simulink model "CraneController"  (R2020b)
settings: Solver=ode45  StartTime=0.0  StopTime=10  MaxStep=1e-5  RelTol=1e-4
values from neighbouring files (symbols this model uses):
  c1 = -3    [ThongSo.m]    (also in ThongSo_Change.m)
  c2 = -3    [ThongSo.m]    (also in ThongSo_Change.m)
  c3 = 10.3    [ThongSo.m]    (also in ThongSo_Change.m)
  c4 = 1    [ThongSo.m]    (also in ThongSo_Change.m)
  eta = 0.05    [ThongSo.m]    (also in ThongSo_Change.m)
  g = 9.81    [ThongSo.m]    (also in ThongSo_Change.m)
  L = 0.305    [ThongSo.m]    (also in ThongSo_Change.m = 0.8)
  M = 1    [ThongSo.m]    (also in ThongSo_Change.m = 5)
  m = 0.8    [ThongSo.m]    (also in ThongSo_Change.m = 1.5)
  tau = 4    [ThongSo.m]    (also in ThongSo_Change.m)
  theta0 = 0    [ThongSo.m]    (also in ThongSo_Change.m)
  theta0_dot = 0    [ThongSo.m]    (also in ThongSo_Change.m)
  theta0_dotdot = 0    [ThongSo.m]    (also in ThongSo_Change.m)
  thetad = 0    [ThongSo.m]    (also in ThongSo_Change.m)
  thetad_dot = 0    [ThongSo.m]    (also in ThongSo_Change.m)
  x0 = 0    [ThongSo.m]    (also in ThongSo_Change.m)
  x0_dot = 0    [ThongSo.m]    (also in ThongSo_Change.m)
  x0_dotdot = 0    [ThongSo.m]    (also in ThongSo_Change.m)
  xd = 1    [ThongSo.m]    (also in ThongSo_Change.m = 2)
  xd_dot = 0    [ThongSo.m]    (also in ThongSo_Change.m)
libraries: powerlib x1
settings Model: Creator=chemi  LastModifiedBy=chemi
settings SolverCC: ZeroCrossAlgorithm=Adaptive
settings DebuggingCC: IgnoredZcDiagnostic=none

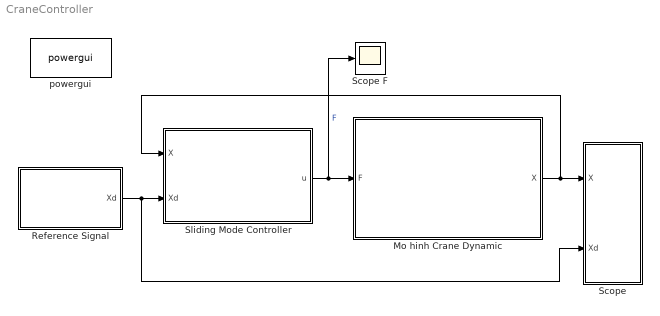
== system CraneController ==
  Mo hinh Crane Dynamic : Subsystem
  Reference Signal : Subsystem
  Scope : Subsystem
  Scope F : Scope
  Sliding Mode Controller : Subsystem
  powergui : powerlib/powergui  Priority=1  SimulationMode=Continuous  SampleTime=50e-6  frequency=60  Iterations=50  frequencyindice=60  Pbase=100e6  ErrMax=1e-4  UnitsV=kV  UnitsW=MW  buscounter=0  FunctionMessages=off  echomessages=off  EnableUseOfTLC=off  CurrentSourceSwitches=off  DisableSnubberDevices=off  DisableRonSwitches=off  DisableVfSwitches=off  DisplayEquations=off  AutomaticDiscreteSolvers=off  SolverType=Tustin/Backward Euler (TBE)  Interpol=off  ExternalGateDelay=off  methode=off  Ts=100  x0status=blocks  SPID=on  SwTol=0  HookPort=off  NonlinearTolerance=1e-4  nMaxIteration=100  ContinueOnMaxIteration=off  RestoreLinks=warning  ResistiveCurrentMeasurement=off  Frange=[0:2:500]  Ylog=off  Xlog=on  ShowGrid=off  save=off  variable=ZData  structure=0  ZoomFFT=off  StartTime=0.0  cycles=1  DisplayStyle=1  fundamental=60  FreqAxis=off  MaxFrequency=1000  frequencyindicesteady=1  RmsSteady=1  display=off
  wires:
  Reference Signal/1(Xd) -> Scope/2(Xd), Sliding Mode Controller/2(Xd)
  Sliding Mode Controller/1(u) -> Scope F/1, Mo hinh Crane Dynamic/1(F)  "F"
  Mo hinh Crane Dynamic/1(X) -> Sliding Mode Controller/1(X), Scope/1(X)

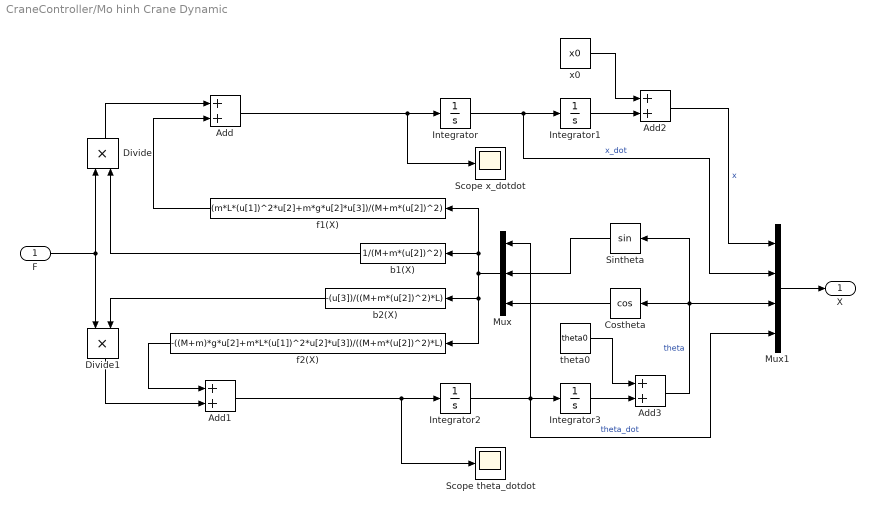
== system CraneController/Mo hinh Crane Dynamic ==
  F : Inport
  Add{,1..3} (4 alike) : Sum
  Costheta : Trigonometry  Operator=cos
  Divide : Product  Inputs=**
  Divide1 : Product  Inputs=**
  Integrator : Integrator  InitialCondition=x0_dotdot
  Integrator1 : Integrator  InitialCondition=x0_dot
  Integrator2 : Integrator  InitialCondition=theta0_dotdot
  Integrator3 : Integrator  InitialCondition=theta0_dot
  Mux : Mux  Inputs=3
  Mux1 : Mux
  Scope theta_dotdot : Scope
  Scope x_dotdot : Scope
  Sintheta : Trigonometry
  b1(X) : Fcn  Expr=1/(M+m*(u[2])^2)
  b2(X) : Fcn  Expr=-(u[3])/((M+m*(u[2])^2)*L)
  f1(X) : Fcn  Expr=(m*L*(u[1])^2*u[2]+m*g*u[2]*u[3])/(M+m*(u[2])^2)
  f2(X) : Fcn  Expr=-((M+m)*g*u[2]+m*L*(u[1])^2*u[2]*u[3])/((M+m*(u[2])^2)*L)
  theta0 : Constant  Value=theta0
  x0 : Constant  Value=x0
  X : Outport
  wires:
  Integrator1/1 -> Add2/2
  Integrator/1 -> Mux1/2, Integrator1/1  "x_dot"
  Integrator2/1 -> Mux1/4, Mux/1, Integrator3/1  "theta_dot"
  F/1 -> Divide/1, Divide1/1
  Mux/1 -> f1(X)/1, b1(X)/1, b2(X)/1, f2(X)/1
  Add/1 -> Scope x_dotdot/1, Integrator/1
  b1(X)/1 -> Divide/2
  Add1/1 -> Scope theta_dotdot/1, Integrator2/1
  f2(X)/1 -> Add1/1
  Divide1/1 -> Add1/2
  b2(X)/1 -> Divide1/2
  Divide/1 -> Add/1
  f1(X)/1 -> Add/2
  x0/1 -> Add2/1
  Integrator3/1 -> Add3/2
  theta0/1 -> Add3/1
  Add3/1 -> Mux1/3, Sintheta/1, Costheta/1  "theta"
  Sintheta/1 -> Mux/2
  Costheta/1 -> Mux/3
  Add2/1 -> Mux1/1  "x"
  Mux1/1 -> X/1

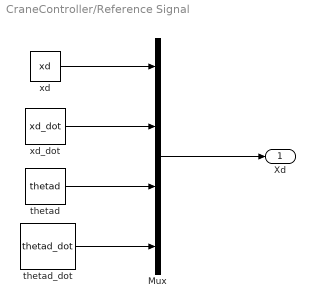
== system CraneController/Reference Signal ==
  Mux : Mux
  thetad : Constant  Value=thetad
  thetad_dot : Constant  Value=thetad_dot
  xd : Constant  Value=xd
  xd_dot : Constant  Value=xd_dot
  Xd : Outport
  wires:
  Mux/1 -> Xd/1
  thetad_dot/1 -> Mux/4
  xd/1 -> Mux/1
  xd_dot/1 -> Mux/2
  thetad/1 -> Mux/3

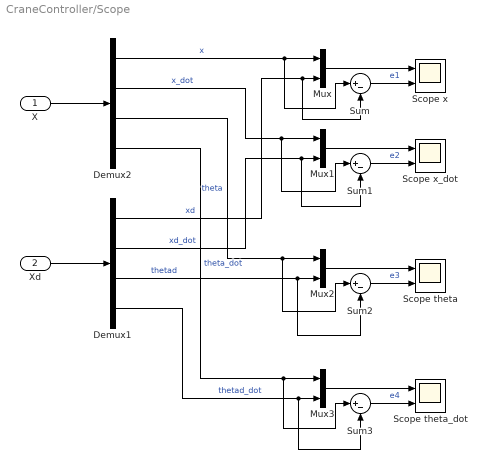
== system CraneController/Scope ==
  X : Inport
  Xd : Inport  Port=2
  Demux1 : Demux
  Demux2 : Demux
  Mux{,1..3} (4 alike) : Mux  Inputs=2
  Scope theta : Scope  NumInputPorts=2
  Scope theta_dot : Scope  NumInputPorts=2
  Scope x : Scope  NumInputPorts=2
  Scope x_dot : Scope  NumInputPorts=2
  Sum{,1..3} (4 alike) : Sum  Inputs=|+-
  wires:
  Mux/1 -> Scope x/1
  X/1 -> Demux2/1
  Xd/1 -> Demux1/1
  Demux2/1 -> Sum/1, Mux/1  "x"
  Demux1/1 -> Sum/2, Mux/2  "xd"
  Sum/1 -> Scope x/2  "e1"
  Demux2/2 -> Mux1/1, Sum1/1  "x_dot"
  Demux1/2 -> Mux1/2, Sum1/2  "xd_dot"
  Mux1/1 -> Scope x_dot/1
  Sum1/1 -> Scope x_dot/2  "e2"
  Demux2/3 -> Sum2/1, Mux2/1  "theta"
  Demux1/3 -> Sum2/2, Mux2/2  "thetad"
  Mux2/1 -> Scope theta/1
  Sum2/1 -> Scope theta/2  "e3"
  Demux2/4 -> Sum3/1, Mux3/1  "theta_dot"
  Demux1/4 -> Sum3/2, Mux3/2  "thetad_dot"
  Mux3/1 -> Scope theta_dot/1
  Sum3/1 -> Scope theta_dot/2  "e4"

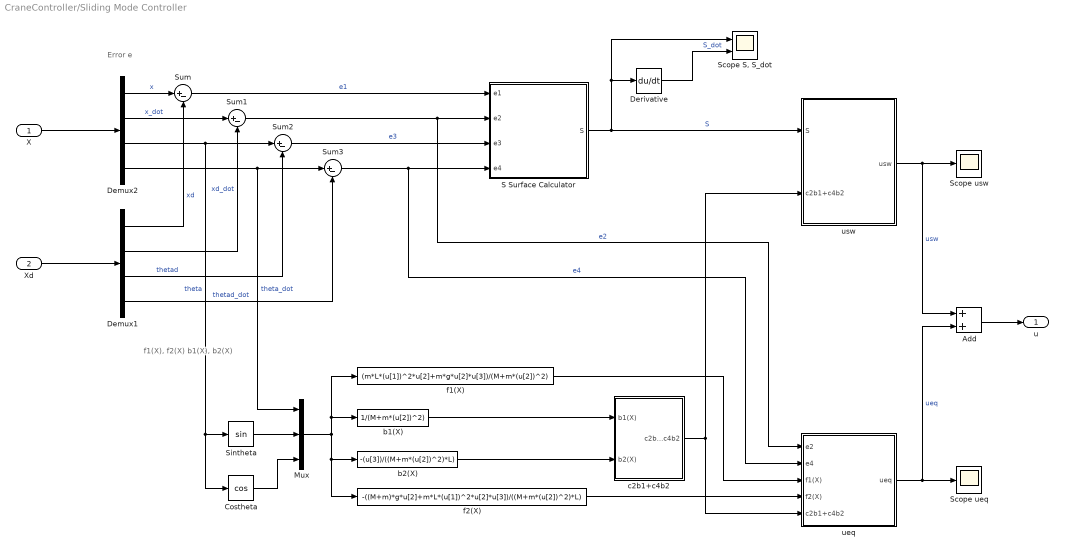
== system CraneController/Sliding Mode Controller ==
  note: Error e
  note: f1(X), f2(X)
      | b1(X), b2(X)
  X : Inport
  Xd : Inport  Port=2
  Add : Sum
  Costheta : Trigonometry  Operator=cos
  Demux1 : Demux
  Demux2 : Demux
  Derivative : Derivative
  Mux : Mux  Inputs=3
  S Surface Calculator : Subsystem
  "Scope S, S_dot" : Scope  NumInputPorts=2
  Scope ueq : Scope
  Scope usw : Scope
  Sintheta : Trigonometry
  Sum{,1..3} (4 alike) : Sum  Inputs=|+-
  b1(X) : Fcn  Expr=1/(M+m*(u[2])^2)
  b2(X) : Fcn  Expr=-(u[3])/((M+m*(u[2])^2)*L)
  c2b1+c4b2 : Subsystem
  f1(X) : Fcn  Expr=(m*L*(u[1])^2*u[2]+m*g*u[2]*u[3])/(M+m*(u[2])^2)
  f2(X) : Fcn  Expr=-((M+m)*g*u[2]+m*L*(u[1])^2*u[2]*u[3])/((M+m*(u[2])^2)*L)
  ueq : Subsystem
  usw : Subsystem
  u : Outport
  wires:
  Sum3/1 -> ueq/2(e4), S Surface Calculator/4(e4)  "e4"
  Sum2/1 -> S Surface Calculator/3(e3)  "e3"
  Sum/1 -> S Surface Calculator/1(e1)  "e1"
  Demux1/2 -> Sum1/2  "xd_dot"
  Demux2/1 -> Sum/1  "x"
  Demux1/4 -> Sum3/2  "thetad_dot"
  X/1 -> Demux2/1
  Xd/1 -> Demux1/1
  Demux1/3 -> Sum2/2  "thetad"
  Demux1/1 -> Sum/2  "xd"
  Sum1/1 -> ueq/1(e2), S Surface Calculator/2(e2)  "e2"
  Mux/1 -> b2(X)/1, f2(X)/1, f1(X)/1, b1(X)/1
  Sintheta/1 -> Mux/2
  Costheta/1 -> Mux/3
  Demux2/4 -> Mux/1, Sum3/1  "theta_dot"
  Demux2/2 -> Sum1/1  "x_dot"
  Demux2/3 -> Sum2/1, Sintheta/1, Costheta/1  "theta"
  S Surface Calculator/1(S) -> "Scope S, S_dot"/1, Derivative/1, usw/1(S)  "S"
  b1(X)/1 -> c2b1+c4b2/1(b1(X))
  b2(X)/1 -> c2b1+c4b2/2(b2(X))
  c2b1+c4b2/1(c2b1+c4b2) -> ueq/5(c2b1+c4b2), usw/2(c2b1+c4b2)
  f1(X)/1 -> ueq/3(f1(X))
  f2(X)/1 -> ueq/4(f2(X))
  Add/1 -> u/1
  usw/1(usw) -> Scope usw/1, Add/1  "usw"
  ueq/1(ueq) -> Scope ueq/1, Add/2  "ueq"
  Derivative/1 -> "Scope S, S_dot"/2  "S_dot"

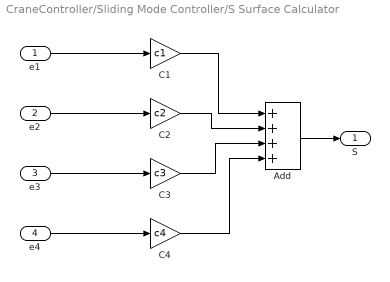
== system CraneController/Sliding Mode Controller/S Surface Calculator ==
  e1 : Inport
  e2 : Inport  Port=2
  e3 : Inport  Port=3
  e4 : Inport  Port=4
  Add : Sum  Inputs=++++
  C1 : Gain  Gain=c1
  C2 : Gain  Gain=c2
  C3 : Gain  Gain=c3
  C4 : Gain  Gain=c4
  S : Outport
  wires:
  e3/1 -> C3/1
  e2/1 -> C2/1
  e4/1 -> C4/1
  e1/1 -> C1/1
  Add/1 -> S/1
  C2/1 -> Add/2
  C3/1 -> Add/3
  C4/1 -> Add/4
  C1/1 -> Add/1

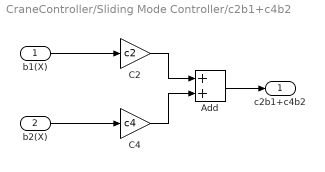
== system CraneController/Sliding Mode Controller/c2b1+c4b2 ==
  b1(X) : Inport
  b2(X) : Inport  Port=2
  Add : Sum
  C2 : Gain  Gain=c2
  C4 : Gain  Gain=c4
  c2b1+c4b2 : Outport
  wires:
  C4/1 -> Add/2
  Add/1 -> c2b1+c4b2/1
  b1(X)/1 -> C2/1
  C2/1 -> Add/1
  b2(X)/1 -> C4/1

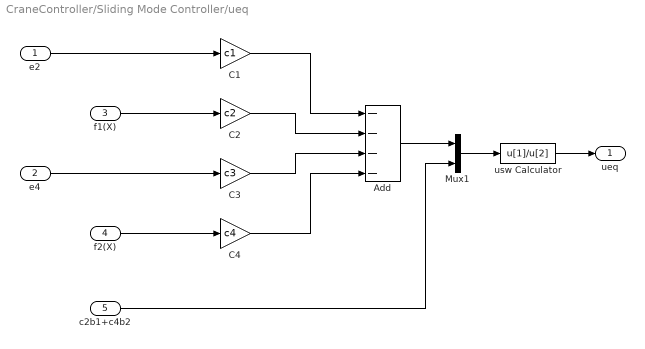
== system CraneController/Sliding Mode Controller/ueq ==
  e2 : Inport
  e4 : Inport  Port=2
  f1(X) : Inport  Port=3
  f2(X) : Inport  Port=4
  c2b1+c4b2 : Inport  Port=5
  Add : Sum  Inputs=----
  C1 : Gain  Gain=c1
  C2 : Gain  Gain=c2
  C3 : Gain  Gain=c3
  C4 : Gain  Gain=c4
  Mux1 : Mux  Inputs=2
  usw Calculator : Fcn  Expr=u[1]/u[2]
  ueq : Outport
  wires:
  Add/1 -> Mux1/1
  Mux1/1 -> usw Calculator/1
  c2b1+c4b2/1 -> Mux1/2
  usw Calculator/1 -> ueq/1
  C4/1 -> Add/4
  C3/1 -> Add/3
  C2/1 -> Add/2
  C1/1 -> Add/1
  e2/1 -> C1/1
  f1(X)/1 -> C2/1
  f2(X)/1 -> C4/1
  e4/1 -> C3/1

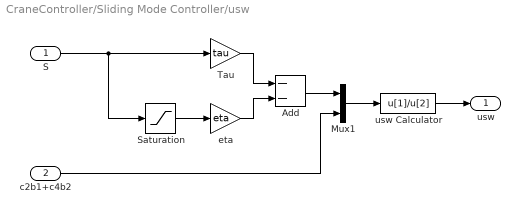
== system CraneController/Sliding Mode Controller/usw ==
  S : Inport
  c2b1+c4b2 : Inport  Port=2
  Add : Sum  Inputs=--
  Mux1 : Mux  Inputs=2
  Saturation : Saturate  UpperLimit=1  LowerLimit=-1
  Tau : Gain  Gain=tau
  eta : Gain  Gain=eta
  usw Calculator : Fcn  Expr=u[1]/u[2]
  usw : Outport
  wires:
  Saturation/1 -> eta/1
  S/1 -> Saturation/1, Tau/1
  Add/1 -> Mux1/1
  Tau/1 -> Add/1
  eta/1 -> Add/2
  Mux1/1 -> usw Calculator/1
  usw Calculator/1 -> usw/1
  c2b1+c4b2/1 -> Mux1/2
